simulink model "weak_feeder_ieee"  (R2024a)
settings: Solver=VariableStepAuto  StartTime=0.0  StopTime=0.5  RelTol=1e-3
libraries: spsThreePhaseParallelRLCLoadLib x9, spsThreePhaseSeriesRLCBranchLib x8, spsThreePhaseDynamicLoadLib x5, spsThreePhaseVIMeasurementLib x2, spsRMSLib x2, spsThreePhaseSourceLib x1, dspstat3 x1, spspowerguiLib x1
settings Model: Creator=Apple  LastModifiedBy=Apple

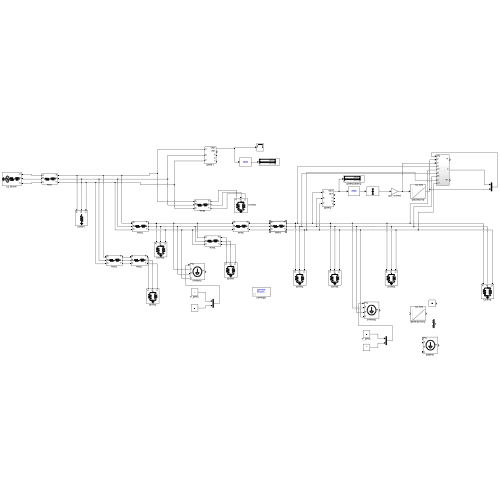
[thumbnail: Simulink's stored preview of the top-level diagram]
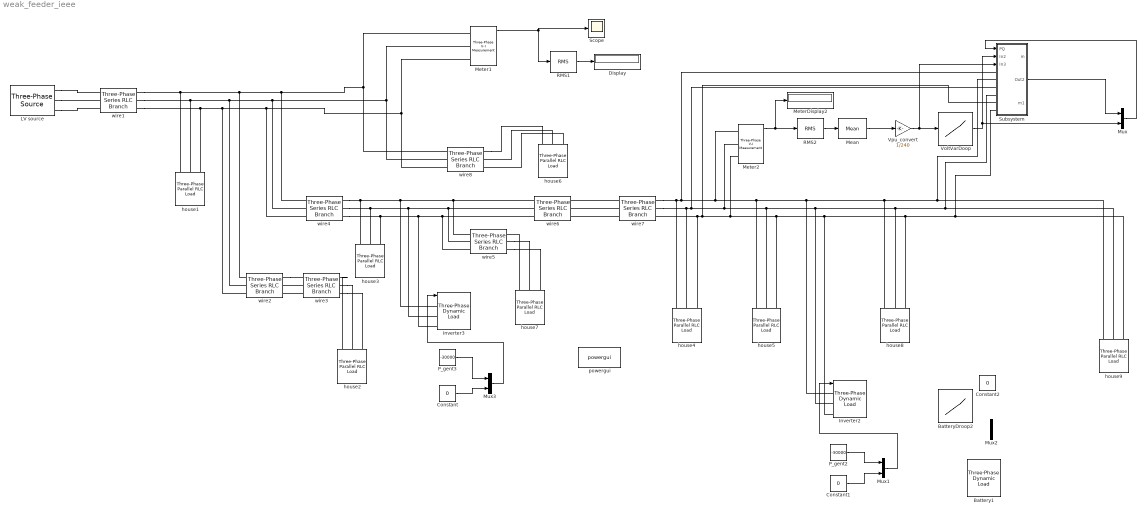
== system weak_feeder_ieee ==
  Battery1 : spsThreePhaseDynamicLoadLib/Three-Phase Dynamic Load  NominalVoltage=[415 50]  ActiveReactivePowers=[0 0]  PositiveSequence=[0.994 -11.8]  ExternalControl=on  NpNq=[1.3 2]  TimeConstants="[0  0  0  0]"  MinimumVoltage=0.7  Tfilter=1e-4  LoadFlowParameters=[4,0,0,0,0]
      settings: LibrarySourceBlock=|
      | sps_lib/Passives/Three-Phase
      | Dynamic Load
  BatteryDroop2 : Lookup_n-D  NumberOfTableDimensions=1  BreakpointsForDimension1=[1.05 1.10]  Table=[0 30000]  ExtrapMethod=Clip  InternalRulePriority=Speed  RndMeth=Simplest
  Constant : Constant  Value=0
  Constant1 : Constant  Value=0
  Constant2 : Constant  Value=0
  Display : Display
  Inverter2 : spsThreePhaseDynamicLoadLib/Three-Phase Dynamic Load  NominalVoltage=[415 50]  ActiveReactivePowers=[50e6 25e6]  PositiveSequence=[0.994 -11.8]  ExternalControl=on  NpNq=[1.3 2]  TimeConstants="[0  0  0  0]"  MinimumVoltage=0.7  Tfilter=1e-4  LoadFlowParameters=[4,0,0,0,0]
      settings: LibrarySourceBlock=|
      | sps_lib/Passives/Three-Phase
      | Dynamic Load
  Inverter3 : spsThreePhaseDynamicLoadLib/Three-Phase Dynamic Load  NominalVoltage=[415 50]  ActiveReactivePowers=[50e6 25e6]  PositiveSequence=[0.994 -11.8]  ExternalControl=on  NpNq=[1.3 2]  TimeConstants="[0  0  0  0]"  MinimumVoltage=0.7  Tfilter=1e-4  LoadFlowParameters=[4,0,0,0,0]
      settings: LibrarySourceBlock=|
      | sps_lib/Passives/Three-Phase
      | Dynamic Load
  LV source : spsThreePhaseSourceLib/Three-Phase Source  InternalConnection=Yg  VoltagePhases=off  Voltage=415  PhaseAngle=0  Voltage_phases=[25e3 25e3 25e3]/sqrt(3)  PhaseAngles_phases=[0 -120 +120]  Frequency=50  NonIdealSource=on  SpecifyImpedance=off  Resistance=0.8929  Inductance=16.58e-3  ShortCircuitLevel=100e6  BaseVoltage=25e3  XRratio=7  BusType=swing  Pref=10e3  Qref=0  Prefabc=[10e3, 10e3, 10e3]  Qrefabc=[0, 0, 0]  Qmin=-inf  Qmax=inf
  Mean : dspstat3/Mean  run=off  InputProcessing=Columns as channels (frame based)  reset_popup=None  directionMode=Entire input  dimension=1  roiEnable=off  roiType=Rectangles  roiPortion=Entire ROI  roiOutput=Individual statistics for each ROI  roiFlag=off  roundingMode=Floor  overflowMode=off  outputDataTypeStr=Inherit: Same as accumulator  outputMin=[]  outputMax=[]  outputLastDataTypeStr=Inherit: Same as accumulator
  Meter1 : spsThreePhaseVIMeasurementLib/Three-Phase V-I Measurement  VoltageMeasurement=phase-to-ground  SetLabelV=off  LabelV=Vabc  Vpu=off  VpuLL=off  CurrentMeasurement=yes  SetLabelI=off  LabelI=Iabc  Ipu=off  Pbase=100e6  Vbase=500e3  OutputType=Complex  PhasorSimulation=off  PSBequivalent=0
  Meter2 : spsThreePhaseVIMeasurementLib/Three-Phase V-I Measurement  VoltageMeasurement=phase-to-ground  SetLabelV=off  LabelV=Vabc  Vpu=off  VpuLL=off  CurrentMeasurement=yes  SetLabelI=off  LabelI=Iabc  Ipu=off  Pbase=100e6  Vbase=500e3  OutputType=Complex  PhasorSimulation=off  PSBequivalent=0
  MeterDisplay2 : Display
  Mux{,1..3} (4 alike) : Mux  Inputs=2
  P_gent2 : Constant  Value=-30000
  P_gent3 : Constant  Value=-30000
  RMS1 : spsRMSLib/RMS  TrueRMS=on  Freq=60  RMSInit=120  Ts=0
  RMS2 : spsRMSLib/RMS  TrueRMS=on  Freq=60  RMSInit=120  Ts=0
  Scope : Scope
  Subsystem : Subsystem
  VoltVarDoop : Lookup_n-D  NumberOfTableDimensions=1  BreakpointsForDimension1=[1.02 1.05]  Table=[0 10000]  ExtrapMethod=Clip  InternalRulePriority=Speed  RndMeth=Simplest
  Vpu_convert : Gain  Gain=1/240
  house1 : spsThreePhaseParallelRLCLoadLib/Three-Phase Parallel RLC Load  LConnTagsString=A|B|C  Configuration=Y (grounded)  NominalVoltage=415  Vabc=[1e3 1e3 1e3]  Vabcp=[1e3 1e3 1e3]  NominalFrequency=50  UnbalancedPower=off  ActivePower=40e3  InductivePower=0  CapacitivePower=0  Pabc=[10e3 9e3 11e3]  QLabc=[100 90 110]  QCabc=[100 90 110]  Pabcp=[10e3 9e3 11e3]  QLabcp=[100 90 110]  QCabcp=[100 90 110]  Measurements=None  LoadType=constant Z
  house2 : spsThreePhaseParallelRLCLoadLib/Three-Phase Parallel RLC Load  LConnTagsString=A|B|C  Configuration=Y (grounded)  NominalVoltage=415  Vabc=[1e3 1e3 1e3]  Vabcp=[1e3 1e3 1e3]  NominalFrequency=50  UnbalancedPower=off  ActivePower=4000  InductivePower=1500  CapacitivePower=0  Pabc=[10e3 9e3 11e3]  QLabc=[100 90 110]  QCabc=[100 90 110]  Pabcp=[10e3 9e3 11e3]  QLabcp=[100 90 110]  QCabcp=[100 90 110]  Measurements=None  LoadType=constant Z
  house3 : spsThreePhaseParallelRLCLoadLib/Three-Phase Parallel RLC Load  LConnTagsString=A|B|C  Configuration=Y (grounded)  NominalVoltage=415  Vabc=[1e3 1e3 1e3]  Vabcp=[1e3 1e3 1e3]  NominalFrequency=50  UnbalancedPower=off  ActivePower=1700  InductivePower=800  CapacitivePower=0  Pabc=[10e3 9e3 11e3]  QLabc=[100 90 110]  QCabc=[100 90 110]  Pabcp=[10e3 9e3 11e3]  QLabcp=[100 90 110]  QCabcp=[100 90 110]  Measurements=None  LoadType=constant Z
  house4 : spsThreePhaseParallelRLCLoadLib/Three-Phase Parallel RLC Load  LConnTagsString=A|B|C  Configuration=Y (grounded)  NominalVoltage=415  Vabc=[1e3 1e3 1e3]  Vabcp=[1e3 1e3 1e3]  NominalFrequency=50  UnbalancedPower=off  ActivePower=2300  InductivePower=1100  CapacitivePower=0  Pabc=[10e3 9e3 11e3]  QLabc=[100 90 110]  QCabc=[100 90 110]  Pabcp=[10e3 9e3 11e3]  QLabcp=[100 90 110]  QCabcp=[100 90 110]  Measurements=None  LoadType=constant Z
  house5 : spsThreePhaseParallelRLCLoadLib/Three-Phase Parallel RLC Load  LConnTagsString=A|B|C  Configuration=Y (grounded)  NominalVoltage=415  Vabc=[1e3 1e3 1e3]  Vabcp=[1e3 1e3 1e3]  NominalFrequency=50  UnbalancedPower=off  ActivePower=1280  InductivePower=600  CapacitivePower=0  Pabc=[10e3 9e3 11e3]  QLabc=[100 90 110]  QCabc=[100 90 110]  Pabcp=[10e3 9e3 11e3]  QLabcp=[100 90 110]  QCabcp=[100 90 110]  Measurements=None  LoadType=constant Z
  house6 : spsThreePhaseParallelRLCLoadLib/Three-Phase Parallel RLC Load  LConnTagsString=A|B|C  Configuration=Y (grounded)  NominalVoltage=415  Vabc=[1e3 1e3 1e3]  Vabcp=[1e3 1e3 1e3]  NominalFrequency=50  UnbalancedPower=off  ActivePower=6000  InductivePower=3000  CapacitivePower=0  Pabc=[10e3 9e3 11e3]  QLabc=[100 90 110]  QCabc=[100 90 110]  Pabcp=[10e3 9e3 11e3]  QLabcp=[100 90 110]  QCabcp=[100 90 110]  Measurements=None  LoadType=constant Z
  house7 : spsThreePhaseParallelRLCLoadLib/Three-Phase Parallel RLC Load  LConnTagsString=A|B|C  Configuration=Y (grounded)  NominalVoltage=415  Vabc=[1e3 1e3 1e3]  Vabcp=[1e3 1e3 1e3]  NominalFrequency=50  UnbalancedPower=off  ActivePower=3400  InductivePower=1700  CapacitivePower=0  Pabc=[10e3 9e3 11e3]  QLabc=[100 90 110]  QCabc=[100 90 110]  Pabcp=[10e3 9e3 11e3]  QLabcp=[100 90 110]  QCabcp=[100 90 110]  Measurements=None  LoadType=constant Z
  house8 : spsThreePhaseParallelRLCLoadLib/Three-Phase Parallel RLC Load  LConnTagsString=A|B|C  Configuration=Y (grounded)  NominalVoltage=415  Vabc=[1e3 1e3 1e3]  Vabcp=[1e3 1e3 1e3]  NominalFrequency=50  UnbalancedPower=off  ActivePower=850  InductivePower=450  CapacitivePower=0  Pabc=[10e3 9e3 11e3]  QLabc=[100 90 110]  QCabc=[100 90 110]  Pabcp=[10e3 9e3 11e3]  QLabcp=[100 90 110]  QCabcp=[100 90 110]  Measurements=None  LoadType=constant Z
  house9 : spsThreePhaseParallelRLCLoadLib/Three-Phase Parallel RLC Load  LConnTagsString=A|B|C  Configuration=Y (grounded)  NominalVoltage=415  Vabc=[1e3 1e3 1e3]  Vabcp=[1e3 1e3 1e3]  NominalFrequency=50  UnbalancedPower=off  ActivePower=1000  InductivePower=500  CapacitivePower=0  Pabc=[10e3 9e3 11e3]  QLabc=[100 90 110]  QCabc=[100 90 110]  Pabcp=[10e3 9e3 11e3]  QLabcp=[100 90 110]  QCabcp=[100 90 110]  Measurements=None  LoadType=constant Z
  powergui : spspowerguiLib/powergui  Priority=1  SimulationMode=Discrete  SampleTime=50e-6  frequency=60  Iterations=50  frequencyindice=50  Pbase=100e6  ErrMax=1e-4  UnitsV=kV  UnitsW=MW  buscounter=0  FunctionMessages=off  echomessages=off  EnableUseOfTLC=off  CurrentSourceSwitches=off  DisableSnubberDevices=off  DisableRonSwitches=off  DisableVfSwitches=off  DisplayEquations=off  AutomaticDiscreteSolvers=off  SolverType=Tustin/Backward Euler (TBE)  Interpol=off  ExternalGateDelay=off  methode=off  Ts=100  x0status=blocks  SPID=on  SwTol=0  HookPort=off  NonlinearTolerance=1e-4  nMaxIteration=100  ContinueOnMaxIteration=off  RestoreLinks=warning  ResistiveCurrentMeasurement=off  Frange=[0:2:500]  Ylog=off  Xlog=on  ShowGrid=off  save=off  variable=ZData  structure=0  ZoomFFT=off  StartTime=0.0  cycles=1  DisplayStyle=1  fundamental=60  FreqAxis=off  MaxFrequency=1000  frequencyindicesteady=1  RmsSteady=1  display=off
  wire1 : spsThreePhaseSeriesRLCBranchLib/Three-Phase Series RLC Branch  LConnTagsString=A|B|C  RConnTagsString=A|B|C  BranchType=RL  Resistance=0.850  Inductance=0.000760  Capacitance=1e-6  Measurements=None
  wire2 : spsThreePhaseSeriesRLCBranchLib/Three-Phase Series RLC Branch  LConnTagsString=A|B|C  RConnTagsString=A|B|C  BranchType=RL  Resistance=0.212  Inductance=0.000189  Capacitance=1e-6  Measurements=None
  wire3 : spsThreePhaseSeriesRLCBranchLib/Three-Phase Series RLC Branch  LConnTagsString=A|B|C  RConnTagsString=A|B|C  BranchType=RL  Resistance=0.042  Inductance=0.0000374  Capacitance=1e-6  Measurements=None
  wire4 : spsThreePhaseSeriesRLCBranchLib/Three-Phase Series RLC Branch  LConnTagsString=A|B|C  RConnTagsString=A|B|C  BranchType=RL  Resistance=0.212  Inductance=0.000189  Capacitance=1e-6  Measurements=None
  wire5 : spsThreePhaseSeriesRLCBranchLib/Three-Phase Series RLC Branch  LConnTagsString=A|B|C  RConnTagsString=A|B|C  BranchType=RL  Resistance=0.127  Inductance=0.000113  Capacitance=1e-6  Measurements=None
  wire6 : spsThreePhaseSeriesRLCBranchLib/Three-Phase Series RLC Branch  LConnTagsString=A|B|C  RConnTagsString=A|B|C  BranchType=RL  Resistance=0.425  Inductance=0.000380  Capacitance=1e-6  Measurements=None
  wire7 : spsThreePhaseSeriesRLCBranchLib/Three-Phase Series RLC Branch  LConnTagsString=A|B|C  RConnTagsString=A|B|C  BranchType=RL  Resistance=0.127  Inductance=0.000113  Capacitance=1e-6  Measurements=None
  wire8 : spsThreePhaseSeriesRLCBranchLib/Three-Phase Series RLC Branch  LConnTagsString=A|B|C  RConnTagsString=A|B|C  BranchType=RL  Resistance=0.850  Inductance=0.000760  Capacitance=1e-6  Measurements=None
  wires:
  Meter1/1 -> Scope/1, RMS1/1
  RMS1/1 -> Display/1
  Meter2/1 -> MeterDisplay2/1, RMS2/1
  RMS2/1 -> Mean/1
  Mean/1 -> Vpu_convert/1
  Vpu_convert/1 -> Subsystem/3(In3), VoltVarDoop/1
  VoltVarDoop/1 -> Subsystem/2(In2), Mux/2
  P_gent3/1 -> Mux3/1
  Constant/1 -> Mux3/2
  Mux3/1 -> Inverter3/1
  P_gent2/1 -> Mux1/1
  Constant1/1 -> Mux1/2
  Mux1/1 -> Inverter2/1
  Mux/1 -> Subsystem/1(PQ)
  Subsystem/2(Out2) -> Mux/1
  connections:
  LV source/RConn2 -- wire1/LConn2
  LV source/RConn1 -- wire1/LConn1
  LV source/RConn3 -- wire1/LConn3
  wire1/RConn1 -- house1/LConn1 -- wire4/LConn1 -- wire8/LConn1 -- Meter1/LConn1 -- wire2/LConn1
  wire1/RConn2 -- house1/LConn2 -- wire4/LConn2 -- wire8/LConn2 -- Meter1/LConn2 -- wire2/LConn2
  wire1/RConn3 -- house1/LConn3 -- wire2/LConn3 -- wire4/LConn3 -- wire8/LConn3 -- Meter1/LConn3
  wire3/LConn3 -- wire2/RConn3
  wire3/LConn2 -- wire2/RConn2
  wire2/RConn1 -- wire3/LConn1
  wire3/RConn1 -- house2/LConn1
  wire3/RConn2 -- house2/LConn2
  wire3/RConn3 -- house2/LConn3
  wire4/RConn1 -- Inverter3/LConn1 -- wire5/LConn1 -- wire6/LConn1 -- house3/LConn1
  wire4/RConn2 -- Inverter3/LConn2 -- wire5/LConn2 -- wire6/LConn2 -- house3/LConn2
  wire4/RConn3 -- Inverter3/LConn3 -- wire5/LConn3 -- wire6/LConn3 -- house3/LConn3
  wire7/LConn1 -- wire6/RConn1
  wire7/LConn2 -- wire6/RConn2
  wire7/LConn3 -- wire6/RConn3
  wire7/RConn2 -- Subsystem/LConn3 -- Meter2/LConn2 -- Inverter2/LConn2 -- Subsystem/LConn4 -- house9/LConn2 -- house8/LConn2 -- house5/LConn2 -- house4/LConn2
  wire8/RConn1 -- house6/LConn1
  house6/LConn2 -- wire8/RConn2
  house6/LConn3 -- wire8/RConn3
  house7/LConn1 -- wire5/RConn1
  wire5/RConn2 -- house7/LConn2
  wire5/RConn3 -- house7/LConn3
  house4/LConn3 -- Subsystem/LConn5 -- Meter2/LConn3 -- Subsystem/LConn6 -- house9/LConn3 -- house8/LConn3 -- Inverter2/LConn3 -- house5/LConn3 -- wire7/RConn3
  wire7/RConn1 -- Subsystem/LConn1 -- Meter2/LConn1 -- Inverter2/LConn1 -- Subsystem/LConn2 -- house9/LConn1 -- house8/LConn1 -- house5/LConn1 -- house4/LConn1

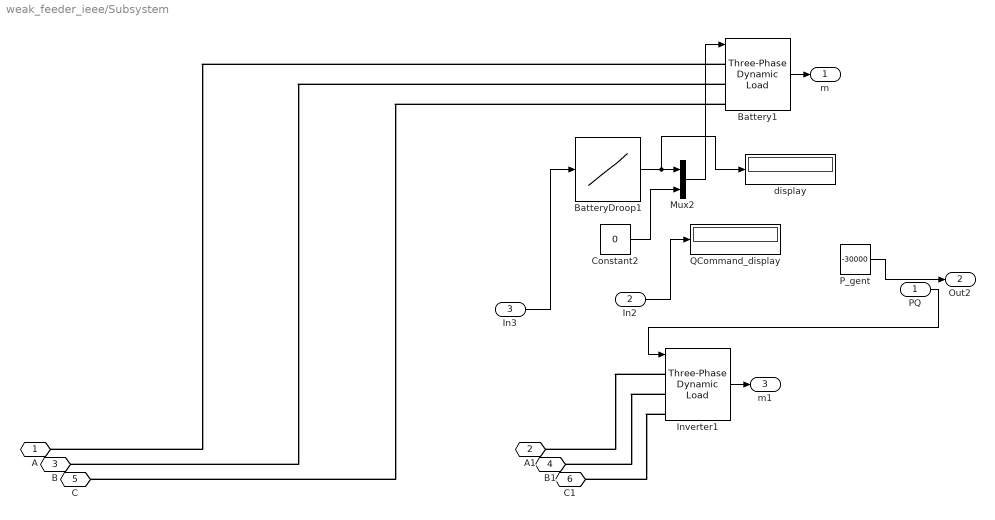
== system weak_feeder_ieee/Subsystem ==
  PQ : Inport
  In2 : Inport  Port=2
  In3 : Inport  Port=3
  Battery1 : spsThreePhaseDynamicLoadLib/Three-Phase Dynamic Load  NominalVoltage=[415 50]  ActiveReactivePowers=[0 0]  PositiveSequence=[0.994 -11.8]  ExternalControl=on  NpNq=[1.3 2]  TimeConstants="[0  0  0  0]"  MinimumVoltage=0.7  Tfilter=1e-4  LoadFlowParameters=[4,0,0,0,0]
      settings: LibrarySourceBlock=|
      | sps_lib/Passives/Three-Phase
      | Dynamic Load
  BatteryDroop1 : Lookup_n-D  NumberOfTableDimensions=1  BreakpointsForDimension1=[1.05 1.10]  Table=[0 30000]  ExtrapMethod=Clip  InternalRulePriority=Speed  RndMeth=Simplest
  Constant2 : Constant  Value=0
  Inverter1 : spsThreePhaseDynamicLoadLib/Three-Phase Dynamic Load  NominalVoltage=[415 50]  ActiveReactivePowers=[50e6 25e6]  PositiveSequence=[0.994 -11.8]  ExternalControl=on  NpNq=[1.3 2]  TimeConstants="[0  0  0  0]"  MinimumVoltage=0.7  Tfilter=1e-4  LoadFlowParameters=[4,0,0,0,0]
      settings: LibrarySourceBlock=|
      | sps_lib/Passives/Three-Phase
      | Dynamic Load
  Mux2 : Mux  Inputs=2
  P_gent : Constant  Value=-30000
  QCommand_display : Display
  display : Display
  A : PMIOPort  Side=Left
  A1 : PMIOPort  Port=2  Side=Left
  B : PMIOPort  Port=3  Side=Left
  B1 : PMIOPort  Port=4  Side=Left
  C : PMIOPort  Port=5  Side=Left
  C1 : PMIOPort  Port=6  Side=Left
  m : Outport
  Out2 : Outport  Port=2
  m1 : Outport  Port=3
  wires:
  P_gent/1 -> Out2/1
  Battery1/1 -> m/1
  PQ/1 -> Inverter1/1
  In3/1 -> BatteryDroop1/1
  In2/1 -> QCommand_display/1
  BatteryDroop1/1 -> display/1, Mux2/1
  Constant2/1 -> Mux2/2
  Mux2/1 -> Battery1/1
  Inverter1/1 -> m1/1
  connections:
  Battery1/LConn3 -- C/RConn1
  Battery1/LConn2 -- B/RConn1
  Inverter1/LConn1 -- A1/RConn1
  Battery1/LConn1 -- A/RConn1
  Inverter1/LConn2 -- B1/RConn1
  Inverter1/LConn3 -- C1/RConn1
